simulink library "tractionControl_lib"  (R2022b)
settings: Solver=VariableStepAuto  StartTime=0.0  StopTime=10.0  RelTol=1e-3
undefined symbols (not defined in the file): raptor_get_param_eval, raptor_xcp_function
libraries: Raptor_lib x10, simulink x2, slpidlib x1
settings Model: Creator=serga  LastModifiedBy=serga

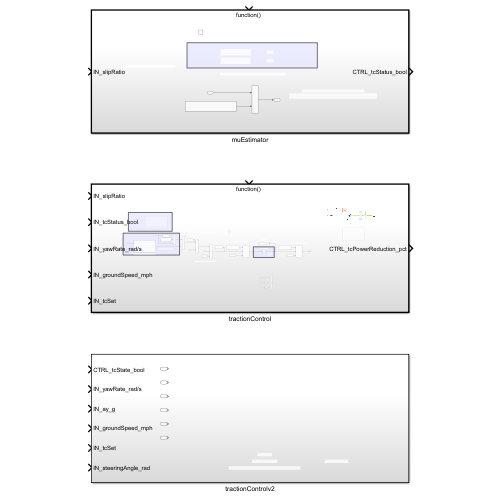
[thumbnail: Simulink's stored preview of the top-level diagram]
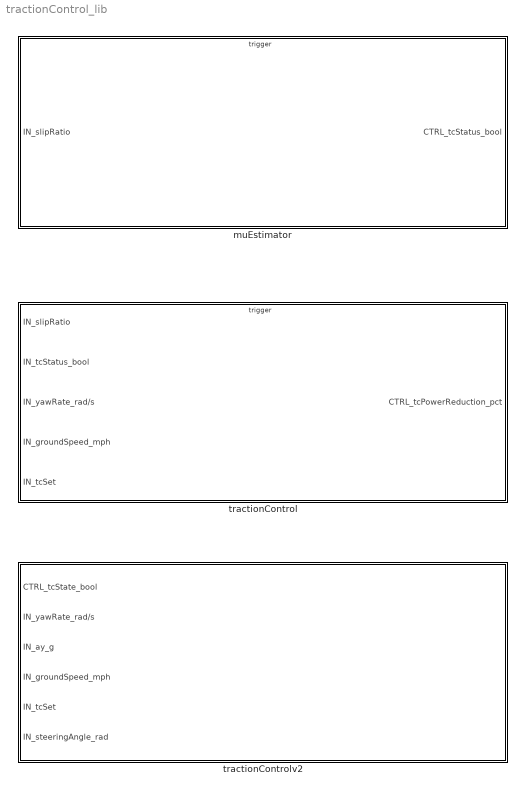
== system tractionControl_lib ==
  muEstimator : Subsystem
  tractionControl : Subsystem  TreatAsAtomicUnit=on
  tractionControlv2 : Subsystem

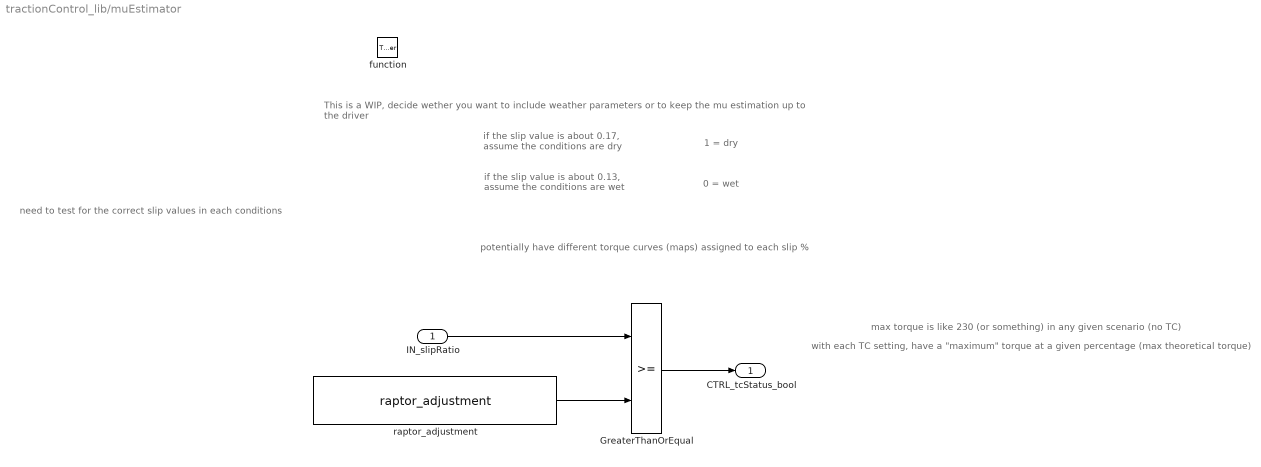
== system tractionControl_lib/muEstimator ==
  note: with each TC setting, have a "maximum" torque at a given percentage (max theoretical torque)
  note: max torque is like 230 (or something) in any given scenario (no TC)
  note: potentially have different torque curves (maps) assigned to each slip %
  note: if the slip value is about 0.17, assume the conditions are dry
  note: 0 = wet
  note: This is a WIP, decide wether you want to include weather parameters or to keep the mu estimation up to the driver
  note: need to test for the correct slip values in each conditions
  note: 1 = dry
  note: if the slip value is about 0.13, assume the conditions are wet
  IN_slipRatio : Inport
  function : TriggerPort  TriggerType=function-call  VariantControl=(inherit)
  GreaterThanOrEqual : RelationalOperator  OutDataTypeStr=boolean  RndMeth=Simplest  InputSameDT=off
  raptor_adjustment : Raptor_lib/Data Storage/raptor_adjustment  paramName='IN_slipThreshold'  nameSource=Parameter  initValue=0.17  dataType=double  storage=Calibration  calDispType=Number  calEnum={'False', 'True'}  calGain=1.0  calOffset=0.0  calMax=inf  calMin=-inf  calFormat='-1'  calUnit=''  calHelp=''  calAccess=1  calFunction=raptor_xcp_function(gcb)  calDispHeaders=off  calColHeaders={'Col1' 'Col2' 'Col3'}  calRowHeaders={'Row1' 'Row2' 'Row3'}
      settings: SourceProductName=Raptor
  CTRL_tcStatus_bool : Outport
  wires:
  IN_slipRatio/1 -> GreaterThanOrEqual/1
  raptor_adjustment/1 -> GreaterThanOrEqual/2
  GreaterThanOrEqual/1 -> CTRL_tcStatus_bool/1

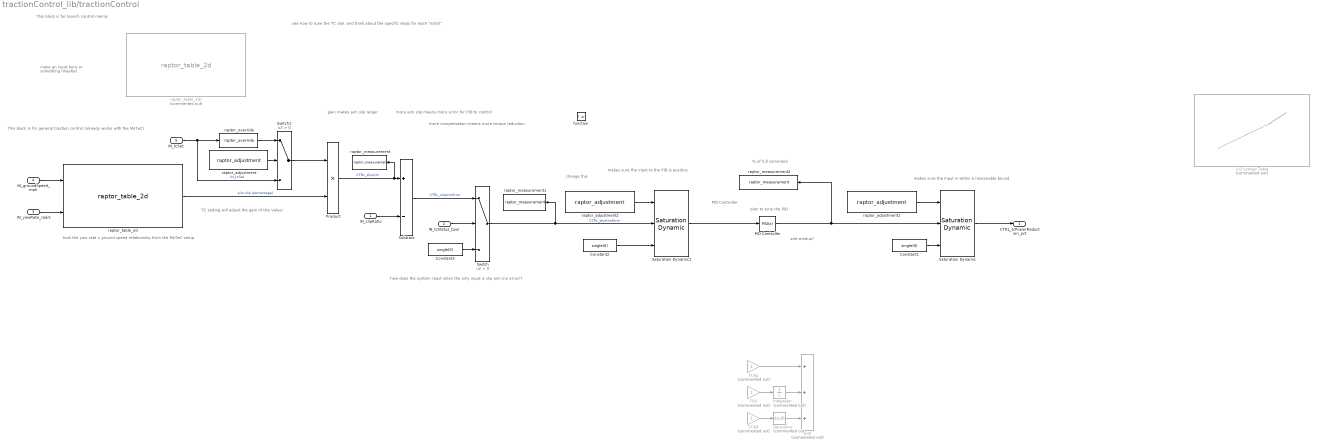
== system tractionControl_lib/tractionControl ==
  note: more compensation means more torque reduction
  note: more aim slip means more error for PID to control
  note: gain makes aim slip larger
  note: anti-windup?
  note: change this
  note: makes sure the input to the PID is positive
  note: % of full command
  note: how does the system react when the only input is slip aim (no error)?
  note: PID Controller
  note: see how to tune the TC dial, and think about the specific steps for each "notch"
  note: makes sure the input is within a reasonable bound
  note: make an input here or something (maybe)
  note: plan to tune the PID
  note: This block is for general traction control (already works with the MoTeC)
  note: This block is for launch control mainly
  note: TC setting will adjust the gain of this value!
  note: took the yaw rate x ground speed relationship from the MoTeC setup
  IN_slipRatio : Inport
  IN_tcStatus_bool : Inport  Port=2
  IN_yawRate_rad/s : Inport  Port=3
  IN_groundSpeed_mph : Inport  Port=4
  IN_tcSet : Inport  Port=5
  function : TriggerPort  TriggerType=function-call  VariantControl=(inherit)
  2-D Lookup Table : Lookup_n-D  Commented=on  LookupTableObject=''  BreakpointsForDimension1=[100 80 70 60 50 40 30 20 10 0]  BreakpointsForDimension2=[-80 -70 -60 -50 -40 -20 0 20 40 50 60 70 80]  BreakpointsForDimension1FirstPoint=10  BreakpointsForDimension2FirstPoint=10  BreakpointsForDimension1Spacing=12  BreakpointsForDimension2Spacing=12  IndexSearchMethod=Evenly spaced points  Table=[5 5.5 6 6.5 7 7.5 8 7.5 7 6.5 6 5.5 5;7 7.5 8 8.5 9 9.5 10 9.5 9 8.5 8 7.5 7;7.5 8 8.5 9 9.5 10 10.5 10 9.5 9 8.5 8 7.5;8 8.5 9 9.5 10 10.5 11 10.5 10 9.5 9 8.5 8;8.5 9 9.5 10 10.5 11 11.5 11 10.5 10 9.5 9 8.5;9 9.5 10 10.5 11 11.5 12 11.5 11 10.5 10 9.5 9;9 9.5 10 10.5 11 11.5 12 11.5 11 10.5 10 9.5 9;9 9.5 10 10.5 11 11.5 12 11.5 11 10.5 10 9.5 9;9 9.5 10 10.5 11 11.5 12 11.5 11 10.5 10 9.5 9;9 9.5 10 10.5 11 11.5 12 11.5 11 10.5 10 9.5 9]  InterpMethod=Flat  DiagnosticForOutOfRangeInput=Error  InternalRulePriority=Speed  RndMeth=Simplest
      settings: InputPortMap=u0,u1
  Add : Sum  Commented=on  Inputs=+++
  Constant1 : Constant  Value=single(0)
  Constant2 : Constant  Value=single(0)
  Constant3 : Constant  Value=single(0)
  Derivative : Derivative  Commented=on
  Integrator : Integrator  Commented=on
  PID Controller : slpidlib/PID Controller  Controller=PID  Form=Parallel  TimeDomain=Discrete-time  UseExternalTs=off  SampleTime=-1  IntegratorMethod=Forward Euler  FilterMethod=Forward Euler  ControllerParametersSource=internal  P=10  I=1  UseKiTs=off  D=10  N=100  UseFilter=off  TunerSelectOption=Transfer Function Based (PID Tuner App)  InitialConditionSource=internal  InitialConditionForIntegrator=0  InitialConditionForFilter=0  DifferentiatorICPrevScaledInput=0  ExternalReset=none  TrackingMode=off  Kt=1  LimitOutput=off  SatLimitsSource=internal  UpperSaturationLimit=inf  LowerSaturationLimit=-inf  LinearizeAsGain=on  AntiWindupMode=none  Kb=1  LimitIntegrator=off  UpperIntegratorSaturationLimit=inf  LowerIntegratorSaturationLimit=-inf  POutMin=[]  POutMax=[]  IOutMin=[]  IOutMax=[]  DOutMin=[]  DOutMax=[]  NOutMin=[]  NOutMax=[]  SumOutMin=[]  SumOutMax=[]  SaturationOutMin=[]  SaturationOutMax=[]  PParamMin=[]  PParamMax=[]  IParamMin=[]  IParamMax=[]  DParamMin=[]  DParamMax=[]  NParamMin=[]  NParamMax=[]  KbParamMin=[]  KbParamMax=[]  KtParamMin=[]  KtParamMax=[]  KbOutMin=[]  KbOutMax=[]  KtOutMin=[]  KtOutMax=[]  IntegratorOutMin=[]  IntegratorOutMax=[]  FilterOutMin=[]  FilterOutMax=[]  SumI1OutMin=[]  SumI1OutMax=[]  SumI2OutMin=[]  SumI2OutMax=[]  SumI3OutMin=[]  SumI3OutMax=[]  SumI4OutMin=[]  SumI4OutMax=[]  SumDOutMin=[]  SumDOutMax=[]  DifferentiatorOutMin=[]  DifferentiatorOutMax=[]  FilterDiffOutCoefMin=[]  FilterDiffOutCoefMax=[]  ReciprocalOutMin=[]  ReciprocalOutMax=[]  SumDenOutMin=[]  SumDenOutMax=[]  SumNumOutMin=[]  SumNumOutMax=[]  DivideOutMin=[]  DivideOutMax=[]  UdiffTsProdOutMin=[]  UdiffTsProdOutMax=[]  NTsProdOutMin=[]  NTsProdOutMax=[]  UintegralTsProdOutMin=[]  UintegralTsProdOutMax=[]  UngainTsProdOutMin=[]  UngainTsProdOutMax=[]  ClampingZeroOutDataTypeStr=Inherit: Inherit via back propagation  ClampingZeroOutMin=[]  ClampingZeroOutMax=[]  FilterDenConstantOutDataTypeStr=Inherit: Inherit via back propagation  FilterDenConstantOutMin=[]  FilterDenConstantOutMax=[]  PCopyOutDataTypeStr=Inherit: Inherit via back propagation  PCopyOutMin=[]  PCopyOutMax=[]  NCopyOutDataTypeStr=Inherit: Inherit via back propagation  NCopyOutMin=[]  NCopyOutMax=[]  IntegratorContinuousStateAttributes=''  IntegratorStateMustResolveToSignalObject=off  IntegratorRTWStateStorageClass=Auto  FilterContinuousStateAttributes=''  FilterStateMustResolveToSignalObject=off  FilterRTWStateStorageClass=Auto  ParallelPVariant=InternalParameters  IdealPVariant=Disabled  IVariant=InternalParameters  DVariant=InternalParameters  IntegratorVariant=Discrete  SatVariant=Disabled  AWVariant=Passthrough  PCopyVariant=Disabled  TRVariant=Disabled  FdbkBlocksVariant=Forward  IdealPFdbkVariant=Disabled  SatFdbkVariant=Disabled  DerivativeFilterVariant=Differentiator  NVariant=Passthrough  NCopyVariant=Disabled_SignalSpec  FilterICVariant=InternalICsDifferentiator  IntegratorICVariant=InternalICs  ExternalResetVariant=Disabled  TRSumVariant=Passthrough  SumFdbkVariant=Disabled  SumVariant=Sum_PID  TsampFilterVariant=InternalTs  TsampNgainVariant=Passthrough  TsampIntegralVariant=Passthrough  ExternalSaturationOutDataTypeStr=Inherit: Same as second input
      settings: AttributesFormatString=|
      | P: %<P>
      | I: %<I>
      | D: %<D>
  Product : Product
  Saturation Dynamic : simulink/Discontinuities/Saturation Dynamic  OutMin=[]  OutMax=[]  OutDataTypeStr=Inherit: Same as second input  OutDataType=fixdt(1, 16)  OutScaling=2^-10  DoSatur=off
  Saturation Dynamic1 : simulink/Discontinuities/Saturation Dynamic  OutMin=[]  OutMax=[]  OutDataTypeStr=Inherit: Same as second input  OutDataType=fixdt(1, 16)  OutScaling=2^-10  DoSatur=off
  Subtract : Sum  Inputs=+-
  Switch : Switch  Criteria=u2 > Threshold  SaturateOnIntegerOverflow=off  InputSameDT=off
  Switch1 : Switch  Criteria=u2 > Threshold  SaturateOnIntegerOverflow=off  InputSameDT=off
  TCKd : Gain  Commented=on
  TCKi : Gain  Commented=on
  TCKp : Gain  Commented=on
  raptor_adjustment : Raptor_lib/Data Storage/raptor_adjustment  paramName='CTRL_tcOverride_bool'  nameSource=Parameter  initValue=0.00  dataType=single  storage=Calibration  calDispType=Number  calEnum={'False', 'True'}  calGain=1.0  calOffset=0.0  calMax=inf  calMin=-inf  calFormat='-1'  calUnit=''  calHelp=''  calAccess=1  calFunction=raptor_xcp_function(gcb)  calDispHeaders=off  calColHeaders={'Col1' 'Col2' 'Col3'}  calRowHeaders={'Row1' 'Row2' 'Row3'}
      settings: SourceProductName=Raptor
  raptor_adjustment1 : Raptor_lib/Data Storage/raptor_adjustment  paramName='CTRL_upperThreshPwrReduction'  nameSource=Parameter  initValue=100  dataType=single  storage=Calibration  calDispType=Number  calEnum={'False', 'True'}  calGain=1.0  calOffset=0.0  calMax=inf  calMin=-inf  calFormat='-1'  calUnit=''  calHelp=''  calAccess=1  calFunction=raptor_xcp_function(gcb)  calDispHeaders=off  calColHeaders={'Col1' 'Col2' 'Col3'}  calRowHeaders={'Row1' 'Row2' 'Row3'}
      settings: SourceProductName=Raptor
  raptor_adjustment2 : Raptor_lib/Data Storage/raptor_adjustment  paramName='CTRL_upperThreshPIDIn'  nameSource=Parameter  initValue=20  dataType=single  storage=Calibration  calDispType=Number  calEnum={'False', 'True'}  calGain=1.0  calOffset=0.0  calMax=inf  calMin=-inf  calFormat='-1'  calUnit=''  calHelp=''  calAccess=1  calFunction=raptor_xcp_function(gcb)  calDispHeaders=off  calColHeaders={'Col1' 'Col2' 'Col3'}  calRowHeaders={'Row1' 'Row2' 'Row3'}
      settings: SourceProductName=Raptor
  raptor_measurement : Raptor_lib/Data Storage/raptor_measurement  paramName='DataName'  nameSource=Input Wire  calDispType=Number  calEnum={'False', 'True'}  calGain=1.0  calOffset=0.0  calMax=inf  calMin=-inf  calFormat='-1'  calUnit=''  calHelp=''  calAccess=1  calFunction=raptor_xcp_function(gcb)  calVisible=on
      settings: SourceProductName=Raptor
  raptor_measurement1 : Raptor_lib/Data Storage/raptor_measurement  paramName='DataName'  nameSource=Input Wire  calDispType=Number  calEnum={'False', 'True'}  calGain=1.0  calOffset=0.0  calMax=inf  calMin=-inf  calFormat='-1'  calUnit=''  calHelp=''  calAccess=1  calFunction=raptor_xcp_function(gcb)  calVisible=on
      settings: SourceProductName=Raptor
  raptor_measurement2 : Raptor_lib/Data Storage/raptor_measurement  paramName='CTRL_tcPowerReduction_pct'  nameSource=Parameter  calDispType=Number  calEnum={'False', 'True'}  calGain=1.0  calOffset=0.0  calMax=inf  calMin=-inf  calFormat='-1'  calUnit=''  calHelp=''  calAccess=1  calFunction=raptor_xcp_function(gcb)  calVisible=on
      settings: SourceProductName=Raptor
  raptor_override : Raptor_lib/Data Storage/raptor_override  paramName='DataName'  nameSource=Input Wire  measurement=None  calDispType=Number  calEnum={'False', 'True'}  calGain=1.0  calOffset=0.0  calMax=inf  calMin=-inf  calFormat='-1'  calUnit=''  calHelp=''  calAccess=1  calFunction="[raptor_xcp_function(gcb) '|'  'Override']"
      settings: SourceProductName=Raptor
  raptor_table_2d : Raptor_lib/Table Lookup/raptor_table_2d  dataName='CTRL_yawRateToAimSlip'  initValue=[5 5.5 6 6.5 7 7.5 8 7.5 7 6.5 6 5.5 5;7 7.5 8 8.5 9 9.5 10 9.5 9 8.5 8 7.5 7;7.5 8 8.5 9 9.5 10 10.5 10 9.5 9 8.5 8 7.5;8 8.5 9 9.5 10 10.5 11 10.5 10 9.5 9 8.5 8;8.5 9 9.5 10 10.5 11 11.5 11 10.5 10 9.5 9 8.5;9 9.5 10 10.5 11 11.5 12 11.5 11 10.5 10 9.5 9;9 9.5 10 10.5 11 11.5 12 11.5 11 10.5 10 9.5 9;9 9.5 10 10.5 11 11.5 12 11.5 11 10.5 10 9.5 9;9 9.5 10 10.5 11 11.5 12 11.5 11 10.5 10 9.5 9;9 9.5 10 10.5 11 11.5 12 11.5 11 10.5 10 9.5 9]  dataType=double  storage=Calibration  initValueX=[-80 -70 -60 -50 -40 -20 0 20 40 50 60 70 80]  initValueY=[100 80 70 60 50 40 30 20 10 0]  dataTypeXY=double  storageXY=Calibration  calVisible=on  showTable=off  calGain=1.0  calOffset=0.0  calMax=Inf  calMin=-Inf  calFormat='-1'  calUnit=''  calHelp=''  showBreakpointX=on  dataNameX=[]  calGainX=1.0  calOffsetX=0.0  calMaxX=Inf  calMinX=-Inf  calFormatX='-1'  calUnitX='rad/s'  calHelpX=''  showBreakpointY=on  dataNameY=[]  calGainY=1.0  calOffsetY=0.0  calMaxY=Inf  calMinY=-Inf  calFormatY='-1'  calUnitY='mph'  calHelpY=''  calAccess=1  calFunction=raptor_xcp_function(gcb)  measureEnable=off  mName=[raptor_get_param_eval(gcb,'dataName'), '_Output']
      settings: SourceProductName=Raptor
  raptor_table_2d1 : Raptor_lib/Table Lookup/raptor_table_2d  Commented=on  dataName='CTRL_accelerometerToAimSlip'  initValue=sqrt([1:11])'*sqrt([1:11])  dataType=double  storage=Calibration  initValueX=[1:11]  initValueY=[1:11]  dataTypeXY=double  storageXY=Calibration  calVisible=on  showTable=off  calGain=1.0  calOffset=0.0  calMax=Inf  calMin=-Inf  calFormat='-1'  calUnit=''  calHelp=''  showBreakpointX=on  dataNameX=[]  calGainX=1.0  calOffsetX=0.0  calMaxX=Inf  calMinX=-Inf  calFormatX='-1'  calUnitX='mps/s'  calHelpX=''  showBreakpointY=on  dataNameY=[]  calGainY=1.0  calOffsetY=0.0  calMaxY=Inf  calMinY=-Inf  calFormatY='-1'  calUnitY='mph'  calHelpY=''  calAccess=1  calFunction=raptor_xcp_function(gcb)  measureEnable=off  mName=[raptor_get_param_eval(gcb,'dataName'), '_Output']
      settings: SourceProductName=Raptor
  CTRL_tcPowerReduction_pct : Outport
  wires:
  Constant3/1 -> Switch/3
  IN_tcStatus_bool/1 -> Switch/2
  IN_slipRatio/1 -> Subtract/2
  IN_groundSpeed_mph/1 -> raptor_table_2d/1
  IN_yawRate_rad/s/1 -> raptor_table_2d/2
  raptor_table_2d/1 -> Product/2  "aim slip (percentage)"
  Product/1 -> raptor_measurement/1, Subtract/1  "CTRL_slipAim"
  Switch/1 -> Saturation Dynamic1/2, raptor_measurement1/1  "CTRL_slipAimError"
  PID Controller/1 -> Saturation Dynamic/2, raptor_measurement2/1
  Saturation Dynamic/1 -> CTRL_tcPowerReduction_pct/1
  Constant1/1 -> Saturation Dynamic/3
  raptor_adjustment1/1 -> Saturation Dynamic/1
  Subtract/1 -> Switch/1  "CTRL_slipAimError"
  Constant2/1 -> Saturation Dynamic1/3
  raptor_adjustment2/1 -> Saturation Dynamic1/1
  Saturation Dynamic1/1 -> PID Controller/1
  Derivative/1 -> Add/3
  TCKd/1 -> Derivative/1
  TCKp/1 -> Add/1
  TCKi/1 -> Integrator/1
  Integrator/1 -> Add/2
  Switch1/1 -> Product/1
  IN_tcSet/1 -> Switch1/3, raptor_override/1  "IN_tcSet"
  raptor_override/1 -> Switch1/1
  raptor_adjustment/1 -> Switch1/2

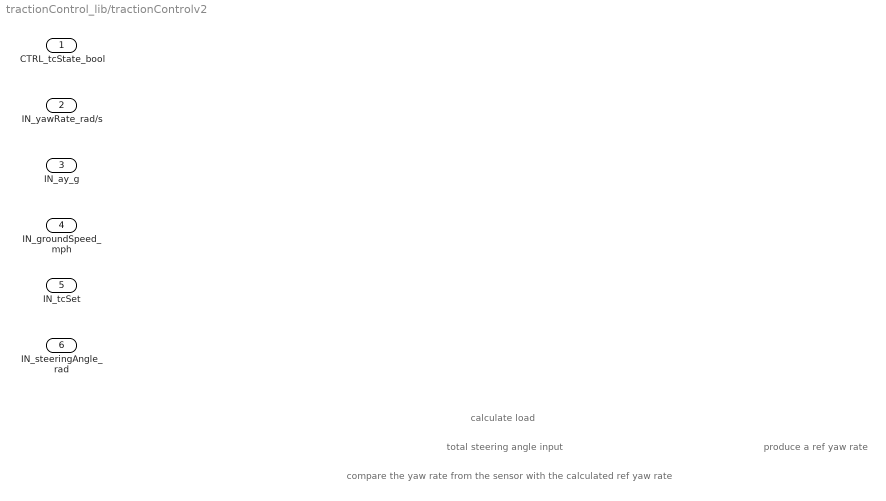
== system tractionControl_lib/tractionControlv2 ==
  note: calculate load
  note: compare the yaw rate from the sensor with the calculated ref yaw rate
  note: produce a ref yaw rate
  note: total steering angle input
  CTRL_tcState_bool : Inport
  IN_yawRate_rad/s : Inport  Port=2
  IN_ay_g : Inport  Port=3
  IN_groundSpeed_mph : Inport  Port=4
  IN_tcSet : Inport  Port=5
  IN_steeringAngle_rad : Inport  Port=6
